simulink model "mag_model_err"  (Simulink 6.2)
settings: Solver=ode45  StartTime=0.0  StopTime=8.0  RelTol=1e-3
settings Model: LastModifiedBy=Martin
settings DebuggingCC: SolverPrmCheckMsg=warning

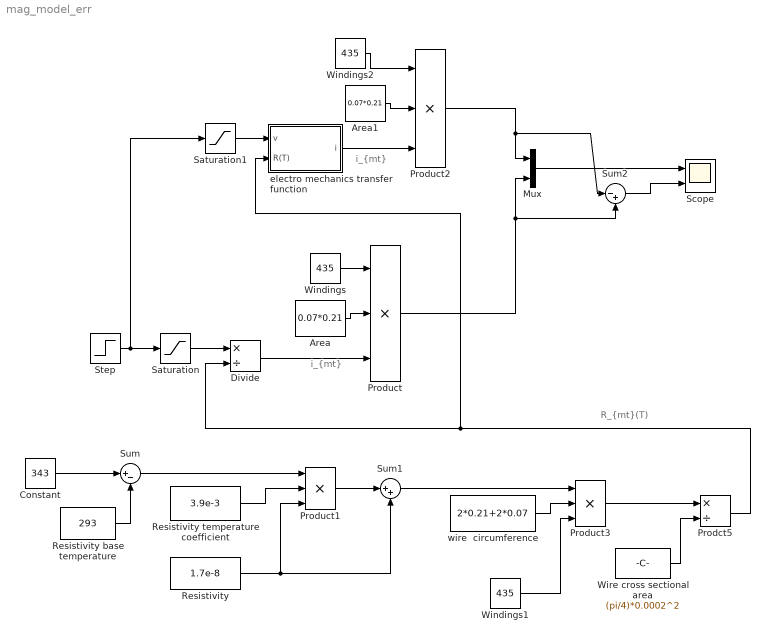
== system mag_model_err ==
  note: R_{mt}(T)
  note: i_{mt}
  note: i_{mt}
  Area : Constant  Value=0.07*0.21
  Area1 : Constant  Value=0.07*0.21
  Constant : Constant  Value=343
  Divide : Product  Inputs=*/  OutScaling=2^-10
  Mux : Mux  Inputs=2
  Prodct5 : Product  Inputs=*/  RndMeth=Zero
  Product{,1..3} (4 alike) : Product  Inputs=3  RndMeth=Zero
  Resistivity : Constant  Value=1.7e-8
  Resistivity base temperature : Constant  Value=293
  Resistivity temperature coefficient : Constant  Value=3.9e-3
  Saturation : Saturate  UpperLimit=5  LowerLimit=-5
  Saturation1 : Saturate  UpperLimit=5  LowerLimit=-5
  Scope : Scope  NumInputPorts=2
      settings: YMin=-5~-5  YMax=5~5  SaveName=mag_induct_err
  Step : Step  After=5  SampleTime=0
  Sum : Sum  Inputs=|+-
  Sum1 : Sum  Inputs=|++
  Sum2 : Sum  Inputs=|-+
  Windings : Constant  Value=435
  Windings1 : Constant  Value=435
  Windings2 : Constant  Value=435
  Wire cross sectional area : Constant  Value=(pi/4)*0.0002^2
  electro mechanics transfer function : Subsystem  AncestorBlock=components_lib/Actuator Emulation/Magnetorquer/electro mechanics transfer function
  wire  circumference : Constant  Value=2*0.21+2*0.07
  wires:
  Prodct5/1 -> Divide/2, electro mechanics transfer function/2(R(T))
  Wire cross sectional area/1 -> Prodct5/2
  Product3/1 -> Prodct5/1
  Windings1/1 -> Product3/3
  wire  circumference/1 -> Product3/2
  Sum1/1 -> Product3/1
  Product1/1 -> Sum1/1
  Resistivity/1 -> Sum1/2, Product1/3
  Sum/1 -> Product1/1
  Resistivity temperature coefficient/1 -> Product1/2
  Constant/1 -> Sum/1
  Resistivity base temperature/1 -> Sum/2
  Step/1 -> Saturation/1, Saturation1/1
  Saturation/1 -> Divide/1
  Divide/1 -> Product/3
  Windings/1 -> Product/1
  Area/1 -> Product/2
  Area1/1 -> Product2/2
  Windings2/1 -> Product2/1
  electro mechanics transfer function/1(i) -> Product2/3
  Saturation1/1 -> electro mechanics transfer function/1(v)
  Product2/1 -> Mux/1, Sum2/1
  Product/1 -> Mux/2, Sum2/2
  Mux/1 -> Scope/1
  Sum2/1 -> Scope/2

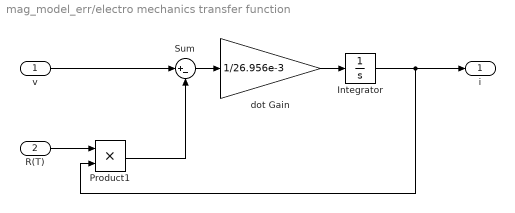
== system mag_model_err/electro mechanics transfer function ==
  v : Inport  Port=1  LatchInput=off
  R(T) : Inport  Port=2  LatchInput=off
  Integrator : Integrator
  Product1 : Product  RndMeth=Zero
  Sum : Sum  Inputs=|+-
  dot Gain : Gain  Gain=1/26.956e-3
  i : Outport
  wires:
  Sum/1 -> dot Gain/1
  dot Gain/1 -> Integrator/1
  Integrator/1 -> Product1/2, i/1
  Product1/1 -> Sum/2
  v/1 -> Sum/1
  R(T)/1 -> Product1/1
